simulink model "test_opt_solver_2015"  (R2015a)
settings: Solver=ode3  SolverMode=SingleTasking  StartTime=0.0  StopTime=10.0  FixedStep=0.002  RelTol=1e-3
settings Model: CovMetricSettings=dwe  CovHtmlReporting=off  covSaveCumulativeToWorkspaceVar=off  CovSaveSingleToWorkspaceVar=off  CovExternalEMLEnable=on  Creator=SUN Runtong  LastModifiedBy=randolf
settings DataIOCC: LimitDataPoints=off  SaveFormat=Dataset
settings OptimizationCC: LocalBlockOutputs=off
settings DebuggingCC: SFUnexpectedBacktrackingDiag=error  SFNoUnconditionalDefaultTransitionDiag=error
settings HardwareCC: ProdBitPerPointer=64  ProdLargestAtomicFloat=Float  ProdIntDivRoundTo=Zero  ProdEndianess=LittleEndian  ProdHWDeviceType=Specified
settings ModelReferenceCC: PropagateSignalLabelsOutOfModel=on
settings SFSimCC: SimUseLocalCustomCode=on
settings RTWCC: Description=TwinCAT Target  SystemTargetFile=TwinCAT.tlc  GenCodeOnly=on  MakeCommand=make_tct  TemplateMakefile=tct_msbuild.tmf  GenerateReport=on  RTWUseLocalCustomCode=on  TargetLang=C++
settings STFCustomTargetCC: TargetLangStandard=C++03 (ISO)  GenerateSampleERTMain=off  CompOptLevelCompliant=on  ERTCustomFileBanners=off  SupportNonInlinedSFcns=on  SupportVariableSizeSignals=off  MATLABClassNameForMDSCustomization=Simulink.SoftwareTarget.TargetSpecificTriggerConfigurationBase  GRTInterface=on  SystemTargetFile=TwinCAT.tlc

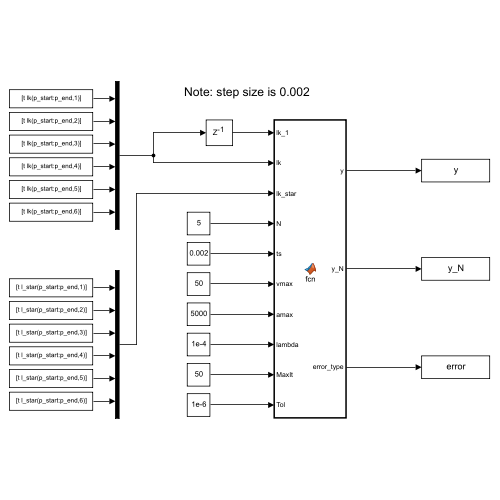
[thumbnail: Simulink's stored preview of the top-level diagram]
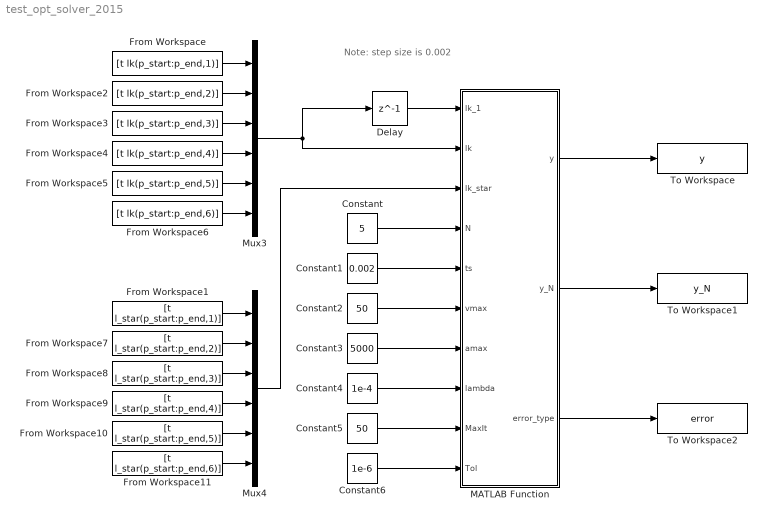
== system test_opt_solver_2015 ==
  note: Note: step size is 0.002
  Constant : Constant  Value=5
  Constant1 : Constant  Value=0.002
  Constant2 : Constant  Value=50
  Constant3 : Constant  Value=5000
  Constant4 : Constant  Value=1e-4
  Constant5 : Constant  Value=50
  Constant6 : Constant  Value=1e-6
  Delay : Delay  DelayLength=1  InitialCondition=0
  From Workspace : FromWorkspace  VariableName=[t lk(p_start:p_end,1)]
  From Workspace1 : FromWorkspace  VariableName=[t l_star(p_start:p_end,1)]
  From Workspace10 : FromWorkspace  VariableName=[t l_star(p_start:p_end,5)]
  From Workspace11 : FromWorkspace  VariableName=[t l_star(p_start:p_end,6)]
  From Workspace2 : FromWorkspace  VariableName=[t lk(p_start:p_end,2)]
  From Workspace3 : FromWorkspace  VariableName=[t lk(p_start:p_end,3)]
  From Workspace4 : FromWorkspace  VariableName=[t lk(p_start:p_end,4)]
  From Workspace5 : FromWorkspace  VariableName=[t lk(p_start:p_end,5)]
  From Workspace6 : FromWorkspace  VariableName=[t lk(p_start:p_end,6)]
  From Workspace7 : FromWorkspace  VariableName=[t l_star(p_start:p_end,2)]
  From Workspace8 : FromWorkspace  VariableName=[t l_star(p_start:p_end,3)]
  From Workspace9 : FromWorkspace  VariableName=[t l_star(p_start:p_end,4)]
  MATLAB Function : MATLAB Function  TreatAsAtomicUnit=on
      settings: PermitHierarchicalResolution=ParametersOnly
  Mux3 : Mux  Inputs=6
  Mux4 : Mux  Inputs=6
  To Workspace : ToWorkspace  VariableName=y  SampleTime=-1
      settings: Save2DSignal=2-D array (concatenate along first dimension)
  To Workspace1 : ToWorkspace  VariableName=y_N  SampleTime=-1
      settings: Save2DSignal=2-D array (concatenate along first dimension)
  To Workspace2 : ToWorkspace  VariableName=error  SampleTime=-1
      settings: Save2DSignal=2-D array (concatenate along first dimension)
  wires:
  Delay/1 -> MATLAB Function/1(lk_1)
  Mux3/1 -> Delay/1, MATLAB Function/2(lk)
  Mux4/1 -> MATLAB Function/3(lk_star)
  Constant/1 -> MATLAB Function/4(N)
  Constant1/1 -> MATLAB Function/5(ts)
  Constant2/1 -> MATLAB Function/6(vmax)
  Constant3/1 -> MATLAB Function/7(amax)
  Constant4/1 -> MATLAB Function/8(lambda)
  Constant5/1 -> MATLAB Function/9(MaxIt)
  Constant6/1 -> MATLAB Function/10(Tol)
  MATLAB Function/1(y) -> To Workspace/1
  MATLAB Function/2(y_N) -> To Workspace1/1
  MATLAB Function/3(error_type) -> To Workspace2/1
  From Workspace6/1 -> Mux3/6
  From Workspace5/1 -> Mux3/5
  From Workspace4/1 -> Mux3/4
  From Workspace3/1 -> Mux3/3
  From Workspace2/1 -> Mux3/2
  From Workspace/1 -> Mux3/1
  From Workspace1/1 -> Mux4/1
  From Workspace7/1 -> Mux4/2
  From Workspace8/1 -> Mux4/3
  From Workspace9/1 -> Mux4/4
  From Workspace11/1 -> Mux4/6
  From Workspace10/1 -> Mux4/5

== matlab function test_opt_solver_2015/MATLAB Function ==
  data: lk_1 input; y output; y_N output; lk input; lk_star input; N input; ts input; vmax input; amax input; lambda input; error_type output; MaxIt input; Tol input
function [y, y_N , error_type] = fcn(lk_1,lk,lk_star,N,ts,vmax,amax,lambda,MaxIt,Tol)
    y = zeros(6,1);
    y_N = zeros(6,1);
    error_type = zeros(6,1);
    %% construct 6 axis mat
    H = diag([2*lambda*ones(1,N-1) 1+lambda]) - 2*lambda*diag([ones(N-1,1)],-1);
    H = 1/2*(H+H');
    Av = eye(N) - diag(ones(N-1,1),-1);
    Aa = eye(N) - 2*diag(ones(N-1,1),-1) + diag(ones(N-2,1),-2);
    A = [Av;
        -Av;
        Aa;
        -Aa];
    bv_base = ts*vmax*ones(2*N,1);
    bv = zeros(2*N,1);
    ba_base = ts^2*amax*ones(2*N,1);
    ba = zeros(2*N,1);
    
    for i = 1:6
        f = [-2*lambda*lk(i)
            zeros(N-2,1)
            -2*lk_star(i)];
        bv = bv_base;
        bv(1) = bv_base(1) + lk(i);
        bv(N+1) = bv_base(N+1) - lk(i); 
        ba = ba_base;
        ba(1) = ba_base(1) - lk_1(i) + 2*lk(i);
        ba(2) = ba_base(2) - lk(i);
        ba(N+1) = ba_base(N+1) + lk_1(i) - 2*lk(i);
        ba(N+2) = ba_base(N+2) + lk(i);
        b = [bv
            ba];
        [x,iter] = MyQP(2*H,f,A,b,[],[],lk(i)*ones(N,1),MaxIt,Tol);
        % if out of planning
        % 1=> true, prime number =>false
        % 2=> size error
        % 3=> null error
        % 5=> iter error
        % 7=> speed error
        % 11=> acc error
        error_type(i) = 1;
        % size error
        if (size(x,1)~=N)
            error_type(i) = error_type(i)*2;
        end
         % null error
        if (sum(isnan(x))>0)
            error_type(i) = error_type(i)*3;
        end
        % iteration
        if (iter>MaxIt)
            error_type(i) = error_type(i)*5;
        end
        % if speed out bound
        if (abs(x(1)-lk(i))>vmax*ts+1e-8)
           error_type(i) = error_type(i)*7; 
        end
        % if acceleration out bound
        if (abs(x(1)-2*lk(i)+lk_1(i))>amax*ts*ts+1e-8)
           error_type(i) = error_type(i)*11; 
        end
        
        if abs(error_type(i) - 1) < 1e-4
            y(i) = x(1);
            y_N(i) = x(N);
        else
            y(i) = lk(i);
        end
    end % end for i=1:6
end
